simulink model "EV_Charger_Design_Sim_2"  (R2021a)
settings: Solver=ode23t  StartTime=0.0  StopTime=1.0  RelTol=1e-3
undefined symbols (not defined in the file): Ion, Lithium
libraries: spsDiodeLib x4, spsIGBTDiodeLib x4, spsMosfetLib x4, eeRmsMeasurement x4, spsSeriesRLCBranchLib x4, spsVoltageMeasurementLib x4, spsCurrentMeasurementLib x3, pid_lib x2, eePowerMeasurement x2, spsACVoltageSourceLib x1, spsBatteryLib x1, spsLinearTransformerLib x1
settings Model: SimulationMode=rapid-accelerator  Creator=Adeboye  LastModifiedBy=Adeboye
settings GRTTargetCC: RTWCAPISignals=on  RTWCAPIParams=on

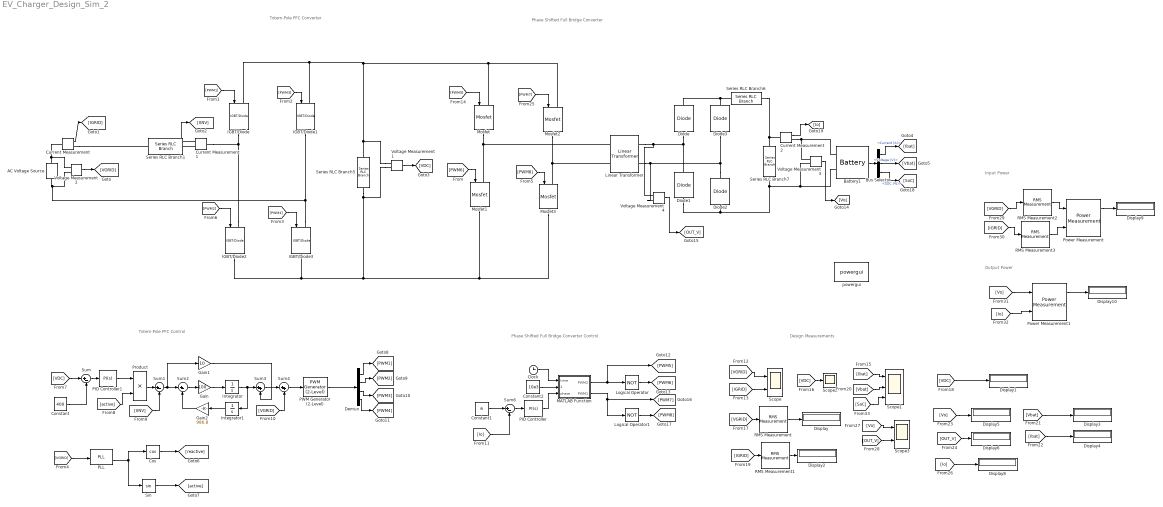
== system EV_Charger_Design_Sim_2 ==
  note: Output Power
  note: Design Measurements
  note: Totem-Pole PFC Control
  note: Phase Shifted Full Bridge Converter Control
  note: Phase Shifted Full Bridge Converter
  note: Totem-Pole PFC Converter
  note: Input Power
  AC Voltage Source : spsACVoltageSourceLib/AC Voltage Source  Amplitude=120*sqrt(2)  Phase=0  Frequency=60  SampleTime=0  Measurements=None  BusType=swing  Pref=10e3  Qref=0  Qmin=-inf  Qmax=+inf
  Battery1 : spsBatteryLib/Battery  BatType=Lithium-Ion  ShowTempParam=off  ThermalPreset=no  ShowAgeParam=off  NomV=340  NomQ=169  SOC=50  Batt_Tr=1  PresetModel=on  MaxQ=169  MinV=255  FullV=395.7556  Dis_rate=73.4783  R=0.020118  Normal_OP=152.8348  expZone="[367.3312      8.303043]"  current=[6.5 13 32.5]  Units=Time  Tci=20  NomT=20  T2=-30  MaxQ2=4.8  FullV2=7.1  Normal_OP2=5.655  expZone2="[6.58           1]"  Rca=0.6  ti=2000  Dp=0  Neq0=0  Tsim=1e6  Ta1=25  Qeol=5.4*0.9  Reol=0.013333*1.2  Char_age=[2.3478, 3]  Dis_age=[2.3478, 10]  N1=1500  N2=10500  N3=1000  N4=1400  Ta2=45  N5=950
  Bus Selector : BusSelector  OutputSignals=Current (A),Voltage (V),SOC (%)
  Clock : Clock
  Constant : Constant  Value=400
  Constant1 : Constant  Value=6
  Constant2 : Constant  Value=10e3
  Cos : Trigonometry  Operator=cos
  Current Measurement : spsCurrentMeasurementLib/Current Measurement  PhasorSimulation=off  OutputType=Complex  PSBequivalent=0
  Current Measurement1 : spsCurrentMeasurementLib/Current Measurement  PhasorSimulation=off  OutputType=Complex  PSBequivalent=0
  Current Measurement2 : spsCurrentMeasurementLib/Current Measurement  PhasorSimulation=off  OutputType=Complex  PSBequivalent=0
  Demux : Demux
  Diode{,1..3} (4 alike) : spsDiodeLib/Diode  Ron=0.001  Lon=0  Vf=0.8  IC=0  UseSnubber=0  Rs=500  Cs=250e-9  Measurements=off
  Display{,1..6,8..10} (10 alike) : Display
  Gain : Gain  Gain=100
  Gain1 : Gain  Gain=10
  Gain2 : Gain  Gain=986.8
  IGBT/Diode{,1..3} (4 alike) : spsIGBTDiodeLib/IGBT//Diode  Ron=1e-3  Rs=1e5  Cs=inf  Measurements=off
  Integrator : Integrator
  Integrator1 : Integrator
  Linear Transformer : spsLinearTransformerLib/Linear Transformer  UNITS=SI  NominalPower=[2400 60 ]  winding1=[400 4.3218e-9 0.45856e-9]  winding2=[410 0.7938e-9 0.084225e-9]  ThreeWindings=off  winding3=[3.15e+05 0.7938 0.084225]  RmLm=[1.0804e+06 2866]  Measurements=None  DataType=on
  Logical Operator : Logic  Operator=NOT  AllPortsSameDT=off  OutDataTypeStr=boolean
  Logical Operator1 : Logic  Operator=NOT  AllPortsSameDT=off  OutDataTypeStr=boolean
  MATLAB Function : MATLAB Function  TreatAsAtomicUnit=on
  Mosfet{,1..3} (4 alike) : spsMosfetLib/Mosfet  Ron=0.1  Lon=0  Rd=0.01  Vfd=0  IC=0  Rs=1e5  Cs=inf  Measurements=off
  PID Controller : pid_lib/PID Controller  Controller=PI  Form=Parallel  TimeDomain=Continuous-time  UseExternalTs=off  SampleTime=-1  IntegratorMethod=Forward Euler  FilterMethod=Forward Euler  ControllerParametersSource=internal  P=50000  I=5000  D=0  UseFilter=on  N=100  TunerSelectOption=Transfer Function Based (PID Tuner App)  InitialConditionSource=internal  InitialConditionForIntegrator=0  InitialConditionForFilter=0  DifferentiatorICPrevScaledInput=0  ExternalReset=none  TrackingMode=off  Kt=1  LimitOutput=on  SatLimitsSource=internal  UpperSaturationLimit=180  LowerSaturationLimit=-inf  LinearizeAsGain=on  AntiWindupMode=none  Kb=1  POutMin=[]  POutMax=[]  IOutMin=[]  IOutMax=[]  DOutMin=[]  DOutMax=[]  NOutMin=[]  NOutMax=[]  SumOutMin=[]  SumOutMax=[]  SaturationOutMin=[]  SaturationOutMax=[]  PParamMin=[]  PParamMax=[]  IParamMin=[]  IParamMax=[]  DParamMin=[]  DParamMax=[]  NParamMin=[]  NParamMax=[]  KbParamMin=[]  KbParamMax=[]  KtParamMin=[]  KtParamMax=[]  KbOutMin=[]  KbOutMax=[]  KtOutMin=[]  KtOutMax=[]  IntegratorOutMin=[]  IntegratorOutMax=[]  FilterOutMin=[]  FilterOutMax=[]  SumI1OutMin=[]  SumI1OutMax=[]  SumI2OutMin=[]  SumI2OutMax=[]  SumI3OutMin=[]  SumI3OutMax=[]  SumI4OutMin=[]  SumI4OutMax=[]  SumDOutMin=[]  SumDOutMax=[]  DifferentiatorOutMin=[]  DifferentiatorOutMax=[]  FilterDiffOutCoefMin=[]  FilterDiffOutCoefMax=[]  ReciprocalOutMin=[]  ReciprocalOutMax=[]  SumDenOutMin=[]  SumDenOutMax=[]  SumNumOutMin=[]  SumNumOutMax=[]  DivideOutMin=[]  DivideOutMax=[]  UdiffTsProdOutMin=[]  UdiffTsProdOutMax=[]  NTsProdOutMin=[]  NTsProdOutMax=[]  UintegralTsProdOutMin=[]  UintegralTsProdOutMax=[]  UngainTsProdOutMin=[]  UngainTsProdOutMax=[]  IntegratorContinuousStateAttributes=''  IntegratorStateMustResolveToSignalObject=off  IntegratorRTWStateStorageClass=Auto  FilterContinuousStateAttributes=''  FilterStateMustResolveToSignalObject=off  FilterRTWStateStorageClass=Auto  ParallelPVariant=InternalParameters  IdealPVariant=Disabled  IVariant=InternalParameters  DVariant=Disabled  IntegratorVariant=Continuous  SatVariant=Enabled  AWVariant=Passthrough  PCopyVariant=Disabled  TRVariant=Disabled  FdbkBlocksVariant=Forward  IdealPFdbkVariant=Disabled  SatFdbkVariant=Disabled  DerivativeFilterVariant=Disabled  NVariant=Disabled  NCopyVariant=Disabled_SignalSpec  FilterICVariant=Disabled  IntegratorICVariant=InternalICs  ExternalResetVariant=Disabled  TRSumVariant=Passthrough  SumFdbkVariant=Disabled  SumVariant=Sum_PI  TsampFilterVariant=InternalTs  TsampNgainVariant=Passthrough  TsampIntegralVariant=Passthrough  ExternalSaturationOutDataTypeStr=Inherit: Same as second input
  PID Controller1 : pid_lib/PID Controller  Controller=PI  Form=Parallel  TimeDomain=Continuous-time  UseExternalTs=off  SampleTime=-1  IntegratorMethod=Forward Euler  FilterMethod=Forward Euler  ControllerParametersSource=internal  P=1  I=10  D=0  UseFilter=on  N=100  TunerSelectOption=Transfer Function Based (PID Tuner App)  InitialConditionSource=internal  InitialConditionForIntegrator=0  InitialConditionForFilter=0  DifferentiatorICPrevScaledInput=0  ExternalReset=none  TrackingMode=off  Kt=1  LimitOutput=off  SatLimitsSource=internal  UpperSaturationLimit=inf  LowerSaturationLimit=-inf  LinearizeAsGain=on  AntiWindupMode=none  Kb=1  POutMin=[]  POutMax=[]  IOutMin=[]  IOutMax=[]  DOutMin=[]  DOutMax=[]  NOutMin=[]  NOutMax=[]  SumOutMin=[]  SumOutMax=[]  SaturationOutMin=[]  SaturationOutMax=[]  PParamMin=[]  PParamMax=[]  IParamMin=[]  IParamMax=[]  DParamMin=[]  DParamMax=[]  NParamMin=[]  NParamMax=[]  KbParamMin=[]  KbParamMax=[]  KtParamMin=[]  KtParamMax=[]  KbOutMin=[]  KbOutMax=[]  KtOutMin=[]  KtOutMax=[]  IntegratorOutMin=[]  IntegratorOutMax=[]  FilterOutMin=[]  FilterOutMax=[]  SumI1OutMin=[]  SumI1OutMax=[]  SumI2OutMin=[]  SumI2OutMax=[]  SumI3OutMin=[]  SumI3OutMax=[]  SumI4OutMin=[]  SumI4OutMax=[]  SumDOutMin=[]  SumDOutMax=[]  DifferentiatorOutMin=[]  DifferentiatorOutMax=[]  FilterDiffOutCoefMin=[]  FilterDiffOutCoefMax=[]  ReciprocalOutMin=[]  ReciprocalOutMax=[]  SumDenOutMin=[]  SumDenOutMax=[]  SumNumOutMin=[]  SumNumOutMax=[]  DivideOutMin=[]  DivideOutMax=[]  UdiffTsProdOutMin=[]  UdiffTsProdOutMax=[]  NTsProdOutMin=[]  NTsProdOutMax=[]  UintegralTsProdOutMin=[]  UintegralTsProdOutMax=[]  UngainTsProdOutMin=[]  UngainTsProdOutMax=[]  IntegratorContinuousStateAttributes=''  IntegratorStateMustResolveToSignalObject=off  IntegratorRTWStateStorageClass=Auto  FilterContinuousStateAttributes=''  FilterStateMustResolveToSignalObject=off  FilterRTWStateStorageClass=Auto  ParallelPVariant=InternalParameters  IdealPVariant=Disabled  IVariant=InternalParameters  DVariant=Disabled  IntegratorVariant=Continuous  SatVariant=Disabled  AWVariant=Passthrough  PCopyVariant=Disabled  TRVariant=Disabled  FdbkBlocksVariant=Forward  IdealPFdbkVariant=Disabled  SatFdbkVariant=Disabled  DerivativeFilterVariant=Disabled  NVariant=Disabled  NCopyVariant=Disabled_SignalSpec  FilterICVariant=Disabled  IntegratorICVariant=InternalICs  ExternalResetVariant=Disabled  TRSumVariant=Passthrough  SumFdbkVariant=Disabled  SumVariant=Sum_PI  TsampFilterVariant=InternalTs  TsampNgainVariant=Passthrough  TsampIntegralVariant=Passthrough  ExternalSaturationOutDataTypeStr=Inherit: Same as second input
  PLL : spsPLLLib/PLL  Fmin=45  Par_Init=[0, 60]  ParK=[180, 3200, 1]  TcD=1e-6  MaxRateChangeFreq=12  FilterCutOffFreq=25  Ts=0  AGC=off
      settings: SourceProductBaseCode=PS
  PWM Generator (2-Level) : spsPWMGenerator2LevelLib/PWM Generator (2-Level)  ModulatorType=Single-phase full-bridge (4 pulses)  ModulatorMode=Unsynchronized  Fc=10000  Pc=90  nF=27  MinMax="[ -1  1 ]"  SamplingTechnique=Natural  ModulatingSignals=off  m=0.8  Freq=60  Phase=0  Ts=0  ShowCarrierOutport=off
  Power Measurement : eePowerMeasurement/Power Measurement  LabelModeActiveChoice=Continuous  F=60  K=[0 1 2 3]  Ts=0
      settings: SourceProductBaseCode=PS
  Power Measurement1 : eePowerMeasurement/Power Measurement  LabelModeActiveChoice=Continuous  F=60  K=[0 1 2 3]  Ts=0
      settings: SourceProductBaseCode=PS
  Product : Product  RndMeth=Zero
  RMS Measurement{,1..3} (4 alike) : eeRmsMeasurement/RMS Measurement  LabelModeActiveChoice=Total  F=60  SpecifyHarmonics=off  K=[0 1 2]  Ts=0
      settings: SourceProductBaseCode=PS
  Scope : Scope  NumInputPorts=2
  Scope1 : Scope  NumInputPorts=3
  Scope2 : Scope
  Scope3 : Scope  NumInputPorts=2
  Series RLC Branch1 : spsSeriesRLCBranchLib/Series RLC Branch  LConnTagsString=__new0  RConnTagsString=__new0  BranchType=L  Resistance=1  Inductance=2.86e-3  SetiL0=off  InitialCurrent=0  Capacitance=1e-6  Setx0=off  InitialVoltage=0  Measurements=None
  Series RLC Branch5 : spsSeriesRLCBranchLib/Series RLC Branch  LConnTagsString=__new0  RConnTagsString=__new0  BranchType=C  Resistance=0.0001  Inductance=1e-3  SetiL0=off  InitialCurrent=0  Capacitance=828.9e-6  Setx0=on  InitialVoltage=400  Measurements=None
  Series RLC Branch6 : spsSeriesRLCBranchLib/Series RLC Branch  LConnTagsString=__new0  RConnTagsString=__new0  BranchType=L  Resistance=0.0001  Inductance=406.7e-6  SetiL0=off  InitialCurrent=0  Capacitance=5600e-6  Setx0=on  InitialVoltage=400  Measurements=None
  Series RLC Branch7 : spsSeriesRLCBranchLib/Series RLC Branch  LConnTagsString=__new0  RConnTagsString=__new0  BranchType=C  Resistance=0.0001  Inductance=20e-3  SetiL0=off  InitialCurrent=0  Capacitance=14.64e-6  Setx0=off  InitialVoltage=400  Measurements=None
  Sin : Trigonometry
  Sum{,1..2,6} (4 alike) : Sum  Inputs=|+-
  Sum3 : Sum  Inputs=|++
  Sum4 : Sum  Inputs=|++
  Voltage Measurement{1..4} (4 alike) : spsVoltageMeasurementLib/Voltage Measurement  PhasorSimulation=off  OutputType=Complex  PSBequivalent=0
  powergui : spspowerguiLib/powergui  SimulationMode=Discrete  SampleTime=1e-6  frequency=60  Iterations=50  frequencyindice=0  Pbase=100e6  ErrMax=1e-4  UnitsV=kV  UnitsW=MW  buscounter=0  FunctionMessages=off  echomessages=off  EnableUseOfTLC=off  CurrentSourceSwitches=off  DisableSnubberDevices=off  DisableRonSwitches=off  DisableVfSwitches=off  DisplayEquations=off  AutomaticDiscreteSolvers=off  SolverType=Tustin/Backward Euler (TBE)  Interpol=off  ExternalGateDelay=off  methode=off  Ts=0  x0status=blocks  SPID=off  SwTol=0  HookPort=off  NonlinearTolerance=1e-4  nMaxIteration=100  ContinueOnMaxIteration=off  RestoreLinks=warning  ResistiveCurrentMeasurement=off  Frange=[0:2:500]  Ylog=off  Xlog=on  ShowGrid=off  save=off  variable=ZData  structure=0  ZoomFFT=on  StartTime=0.0  cycles=1  DisplayStyle=1  fundamental=60  FreqAxis=off  MaxFrequency=1000  frequencyindicesteady=1  RmsSteady=1  display=off
  wires:
  Current Measurement2/1 -> [Io]
  [Io] -> Display8/1
  MATLAB Function/2(PWM1) -> Logical Operator1/1, [PWM7]
  PID Controller/1 -> MATLAB Function/3(phase)
  MATLAB Function/1(PWM2) -> [PWM5], Logical Operator/1
  Voltage Measurement4/1 -> [OUT_V]
  Clock/1 -> MATLAB Function/1(time)
  Constant1/1 -> Sum6/1
  [Io] -> Sum6/2
  Constant2/1 -> MATLAB Function/2(frequency)
  Logical Operator1/1 -> [PWM8]
  [PWM8] -> Mosfet3/1
  Integrator1/1 -> Gain2/1
  Bus Selector/2 -> [Vbat]  "<Voltage (V)>"
  [PWM3] -> IGBT/Diode1/1
  Gain2/1 -> Sum2/2
  RMS Measurement1/1 -> Display2/1
  [VGRID] -> Scope/1
  [PWM7] -> Mosfet2/1
  [Vo] -> Display5/1
  [OUT_V] -> Display6/1
  Sum6/1 -> PID Controller/1
  Bus Selector/1 -> [Ibat]  "<Current (A)>"
  [VDC] -> Sum/1
  Sum2/1 -> Gain/1
  [Vbat] -> Display3/1
  [Ibat] -> Display4/1
  Sum3/1 -> Sum4/1
  [PWM6] -> Mosfet1/1
  Demux/3 -> [PWM3]
  [PWM1] -> IGBT/Diode/1
  [IGRID] -> Scope/2
  [Vbat] -> Scope1/2
  PLL/2 -> Sin/1, Cos/1
  Battery1/1 -> Bus Selector/1
  [VDC] -> Display1/1
  [VGRID] -> PLL/1
  Voltage Measurement2/1 -> [VGRID]
  Demux/4 -> [PWM4]
  Integrator/1 -> Sum3/1, Integrator1/1
  [PWM2] -> IGBT/Diode2/1
  Voltage Measurement3/1 -> [Vo]
  Current Measurement1/1 -> [IINV]
  RMS Measurement/1 -> Display/1
  [IINV] -> Sum1/2
  [VDC] -> Scope2/1
  [IGRID] -> RMS Measurement1/1
  [Ibat] -> Scope1/1
  [PWM4] -> IGBT/Diode3/1
  Cos/1 -> [reactive]
  Sum/1 -> PID Controller1/1
  Sum4/1 -> PWM Generator (2-Level)/1
  [PWM5] -> Mosfet/1
  Gain1/1 -> Sum3/2
  [VGRID] -> Sum4/2
  [active] -> Product/2
  Demux/2 -> [PWM2]
  Product/1 -> Sum1/1
  Demux/1 -> [PWM1]
  Constant/1 -> Sum/2
  Sum1/1 -> Sum2/1, Gain1/1
  Gain/1 -> Integrator/1
  Voltage Measurement1/1 -> [VDC]
  Current Measurement/1 -> [IGRID]
  Logical Operator/1 -> [PWM6]
  PWM Generator (2-Level)/1 -> Demux/1
  [VGRID] -> RMS Measurement/1
  Sin/1 -> [active]
  PID Controller1/1 -> Product/1
  [Vo] -> Power Measurement1/1
  RMS Measurement2/1 -> Power Measurement/1
  Power Measurement1/1 -> Display10/1
  [Io] -> Power Measurement1/2
  [IGRID] -> RMS Measurement3/1
  [VGRID] -> RMS Measurement2/1
  RMS Measurement3/1 -> Power Measurement/2
  [Vo] -> Scope3/1
  [OUT_V] -> Scope3/2
  Power Measurement/1 -> Display9/1
  Bus Selector/3 -> [SoC]  "<SOC (%)>"
  [SoC] -> Scope1/3
  connections:
  Voltage Measurement3/LConn1 -- Battery1/LConn1 -- Current Measurement2/RConn1
  Diode3/RConn1 -- Diode/RConn1 -- Series RLC Branch6/RConn1
  Voltage Measurement3/LConn2 -- Battery1/LConn2 -- Diode1/LConn1 -- Diode2/LConn1 -- Series RLC Branch7/RConn1
  Linear Transformer/RConn1 -- Voltage Measurement4/LConn1 -- Diode1/RConn1 -- Diode/LConn1
  IGBT/Diode3/LConn1 -- Voltage Measurement2/LConn2 -- AC Voltage Source/LConn1 -- IGBT/Diode1/RConn1
  Voltage Measurement1/LConn2 -- Series RLC Branch5/RConn1 -- Mosfet3/RConn1 -- Mosfet1/RConn1 -- IGBT/Diode2/RConn1 -- IGBT/Diode3/RConn1
  Diode2/RConn1 -- Voltage Measurement4/LConn2 -- Linear Transformer/RConn2 -- Diode3/LConn1
  Current Measurement/RConn1 -- Series RLC Branch1/LConn1
  Current Measurement2/LConn1 -- Series RLC Branch7/LConn1 -- Series RLC Branch6/LConn1
  Voltage Measurement1/LConn1 -- Series RLC Branch5/LConn1 -- Mosfet2/LConn1 -- Mosfet/LConn1 -- IGBT/Diode/LConn1 -- IGBT/Diode1/LConn1
  Mosfet2/RConn1 -- Linear Transformer/LConn2 -- Mosfet3/LConn1
  Mosfet/RConn1 -- Linear Transformer/LConn1 -- Mosfet1/LConn1
  Voltage Measurement2/LConn1 -- AC Voltage Source/RConn1 -- Current Measurement/LConn1
  IGBT/Diode2/LConn1 -- IGBT/Diode/RConn1 -- Current Measurement1/LConn1
  Current Measurement1/RConn1 -- Series RLC Branch1/RConn1

== matlab function EV_Charger_Design_Sim_2/MATLAB Function ==
  data: time input; PWM2 output; frequency input; phase input; PWM1 output
function [PWM2, PWM1] = fcn(time, frequency, phase)
T_switching = 1/frequency;
PWM1 = 0;
PWM2 = 0;
x = mod(time,T_switching);
if x < T_switching/2
    PWM1 = 1;
end
t_phi = T_switching*phase/360;
y = mod(time+t_phi, T_switching);
if y < T_switching/2
    PWM2 = 1;
end
